simulink model "lab2_1"  (Simulink 7.9)
settings: Solver=ode45  StartTime=1  StopTime=2  RelTol=1e-3
libraries: simulink x1
settings Model: Creator=Aquirel  LastModifiedBy=Aquirel

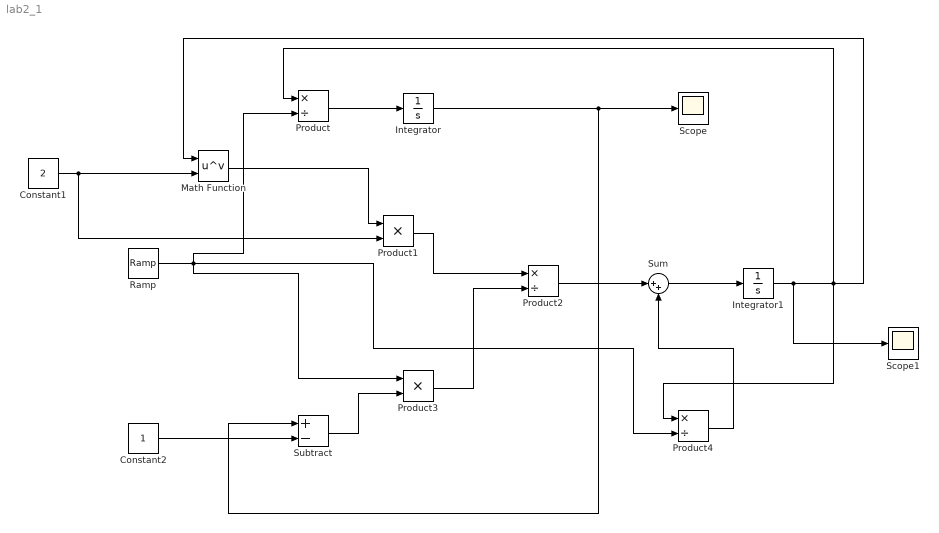
== system lab2_1 ==
  Constant1 : Constant  Value=2
  Constant2 : Constant
  Integrator : Integrator
  Integrator1 : Integrator  InitialCondition=1/3
  Math Function : Math  Operator=pow  SaturateOnIntegerOverflow=on
  Product : Product  Inputs=*/  RndMeth=Zero
  Product1 : Product  Inputs=**  RndMeth=Zero
  Product2 : Product  Inputs=*/  RndMeth=Zero
  Product3 : Product  Inputs=**  RndMeth=Zero
  Product4 : Product  Inputs=*/  RndMeth=Zero
  Ramp : simulink/Sources/Ramp  slope=1  start=0  X0=0
  Scope : Scope
      settings: TimeRange=1  YMin=0  YMax=0.5
  Scope1 : Scope
      settings: YMin=0  YMax=0.5
  Subtract : Sum  Inputs=+-
  Sum : Sum  Inputs=|++
  wires:
  Product/1 -> Integrator/1
  Product1/1 -> Product2/1
  Product3/1 -> Product2/2
  Ramp/1 -> Product/2, Product4/2, Product3/1
  Constant1/1 -> Math Function/2, Product1/2
  Subtract/1 -> Product3/2
  Integrator/1 -> Subtract/1, Scope/1
  Constant2/1 -> Subtract/2
  Product2/1 -> Sum/1
  Math Function/1 -> Product1/1
  Product4/1 -> Sum/2
  Sum/1 -> Integrator1/1
  Integrator1/1 -> Math Function/1, Product/1, Product4/1, Scope1/1
